simulink model "Correlation_Ex5"  (R2025a)
settings: Solver=VariableStepAuto  StartTime=0.0  StopTime=512/100e6  RelTol=1e-3
InitFcn:
  | RTP_F = 40;
  | RTP_G = 24;
undefined symbols (not defined in the file): Correlation_ValidMode, DUT, Full, S, vsva2197, xcvc1902
libraries: visionstatistics x1, aieDSP x1, aieUtilities x1, vmcUtilities x1
settings Model: Creator=sdegala  LastModifiedBy=sdegala
settings ModelReferenceCC: EnableRefExpFcnMdlSchedulingChecks=on
settings RTWCC: GPUComputeCapability=3.5

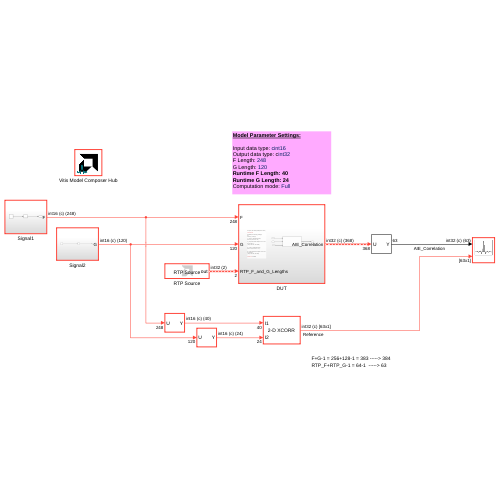
[thumbnail: Simulink's stored preview of the top-level diagram]
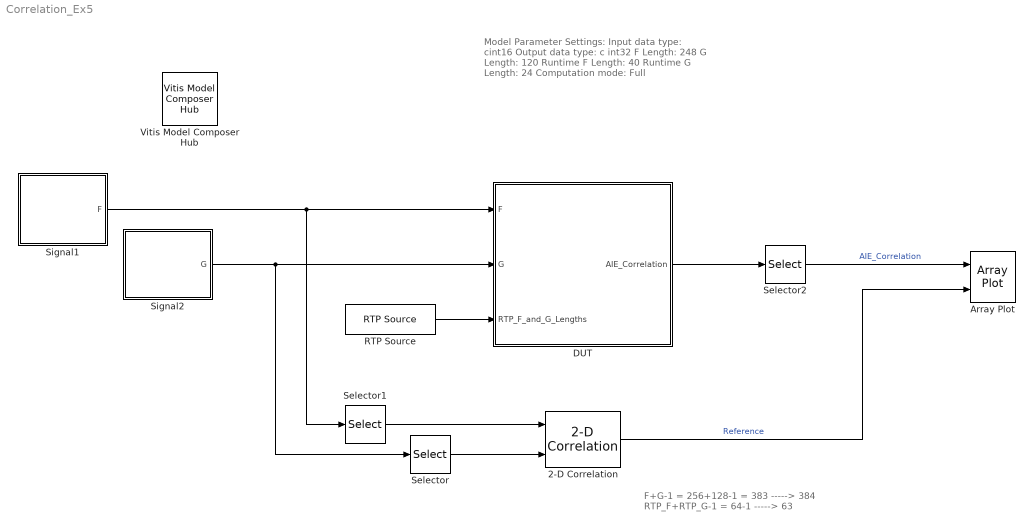
== system Correlation_Ex5 ==
  note: F+G-1 = 256+128-1 = 383 -----> 384
      | RTP_F+RTP_G-1 = 64-1  -----> 63
  note: Model Parameter Settings:
      |
      | Input data type: cint16
      | Output data type: c int32
      | F Length: 248
      | G Length: 120
      | Runtime F Length: 40
      | Runtime G Length: 24
      | Computation mode: Full
  2-D Correlation : visionstatistics/2-D Correlation  outSize=Full  normalize=off  roundingMode=Floor  overflowMode=off  outputMode=Binary point scaling  outputWordLength=32  outputFracLength=0
  Array Plot : ArrayPlot  NumInputPorts=2  WindowPosition=[1138.000000,485.000000,745.000000,420.000000,]  Visible=on  ScopeFrameLocation=window  YLimits=[-15.125 36.125]  ShowLegend=on
  DUT : Subsystem
  RTP Source : aieUtilities/RTP Source  Value=int32([RTP_F,RTP_G]')  SampleTime=-1  OutputForm=Empty
  Selector : Selector  InputPortWidth=120  IndexOptions=Index vector (dialog)  Indices=1:1:RTP_G  OutputSizes=1
  Selector1 : Selector  InputPortWidth=248  IndexOptions=Index vector (dialog)  Indices=1:1:RTP_F  OutputSizes=1
  Selector2 : Selector  InputPortWidth=248+120  IndexOptions=Index vector (dialog)  Indices=1:1:RTP_F+RTP_G-1  OutputSizes=1
  Signal1 : Subsystem
  Signal2 : Subsystem
  Vitis Model Composer Hub : vmcUtilities/Vitis Model Composer Hub  Tag=genX  CodeGeneration=off  SubsystemName=DUT  BlockHierPath=Correlation_ValidMode/DUT  SubsystemType=AIENode  StartColumn=1  NumberOfColumns=1  TargetDirectory=./code  exportDesign=off  analyzeDesign=on  validateDesignOnHw=off  ExportType=AI Engines  IpVendor=xilinx.com  IpLibrary=hls  IpVersion=1.0  IpHWLanguage=Verilog  AieCompilerOptions={}  AieSimulatorOptions={}  CreateTestbench=on  TestbenchStackSize=10  RunRtlSim=off  RunCSim=off  RunAieSim=off  enableSimulationTimeout=on  enableGraphIterations=on  AieSimTimeout=50000  AieGraphIterations=-1  RunAieSimProfiling=off  LaunchVitisAnalyzer=off  PlotOutput=off  RunX86Sim=off  X86SimTimeout=10  GenHwImage=off  GenLibadfXo=off  GenHwValidationCode=off  PlatformType=Not Specified  HwSystemType=Baremetal  HwValidationTarget=hw  ProjDevice=xcvc1902-vsva2197-1LP-e-S  ProjDevicePart=xcvc1902-vsva2197-1LP-e-S  AIEType=AIE  SamplePeriod=-1  ClockFrequency=200  DataPathParallelism=1  xilinxfamily=versalaicore  part=xcvc1902  speed=-1LP-e-S  package=vsva2197  directory=./netlist  testbench=off  incr_netlist=off  synthesis_tool=Vivado  clock_wrapper=Clock Enables  dbl_ovrd=According to Block Masks  dcm_input_clock_period=10  sysclk_period=10  simulink_period=1  eval_field=0  IPInfoJsonString="{\"DUTSubsystemName\":\"DUT\",\"AIESubsystem\":{\"SubsystemName\":\"DUT\",\"TargetDirectory\":\"./code\",\"AIEArrayConfig\":\"Use entire AIE array\",\"StartColumn\":\"0\",\"NumberOfColumns\":\"1\"},\"SubsystemTag\":\"AIENode\"}"  LogFileName=/proj/xhdhdstaff5/sdegala/Head1/HEAD/2025_2_work/AIE_BLOCKS_2025_2/code/model_composer.log  NThreads=4  IPConfigFile=/tmp/vmctmp-11198269997411262707/Correlation_ValidMode_ipconfig.json
  wires:
  Signal1/1(F) -> Selector1/1, DUT/1(F)
  DUT/1(AIE_Correlation) -> Selector2/1
  RTP Source/1 -> DUT/3(RTP_F_and_G_Lengths)
  2-D Correlation/1 -> Array Plot/2  "Reference"
  Selector/1 -> 2-D Correlation/2
  Signal2/1(G) -> DUT/2(G), Selector/1
  Selector1/1 -> 2-D Correlation/1
  Selector2/1 -> Array Plot/1  "AIE_Correlation"

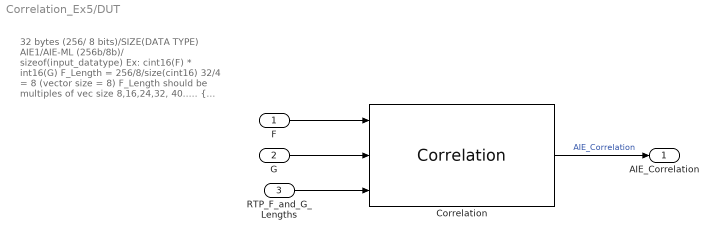
== system Correlation_Ex5/DUT ==
  note: 32 bytes (256/ 8 bits)/SIZE(DATA TYPE)
      |
      | AIE1/AIE-ML
      | (256b/8b)/ sizeof(input_datatype)
      | Ex:
      | cint16(F) * int16(G)
      | F_Length = 256/8/size(cint16)
      | 32/4 = 8 (vector size = 8)
      |
      | F_Length should be multiples of vec size 8,16,24,32, 40.....
      | { range: min-16, max-4096}
      |
      | G_Length = 256/8/size(int16)
      | 32/2 = 16 (vector size = 16)
      |
      | G_Length should be multiples of vec size
      | 16,32,48,64.....
      | { range: min-32, max-256}
      |
      | AIE-MLv2: 512b/8b
  F : Inport
  G : Inport  Port=2
  RTP_F_and_G_Lengths : Inport  Port=3
  Correlation : aieDSP/Correlation  AIE_VARIANT=1  api=0  data_type_f=cint16  data_type_g=cint16  data_type_out=cint32  function_type=0  compute_mode=Full (0)  f_sample_size=248  g_sample_size=120  USE_RTP_VECTOR_LENGTHS=on  num_frames=1  shift_output=0  rnd_mode=Floor  sat_mode=None  no_of_kernels=1  casc_length=1  blockJsonConstraints=[]  blockJsonConstraintsInternal=[]  spec=vmc_corr.json  SerializedMaskParamNames=[]  SerializedMaskParamValues=[]  SerializedMaskParamVisibilities=[]  block_type=Correlation  SerializedMaskParamDataypes=uint|uint|typename|typename|typename|uint|uint|uint|uint|uint|uint|uint|uint|uint|uint|uint  SerializedMaskParamEnumStrArr=0|0|0|0|0|0|Full (0),Same (1),Valid (2)|0|0|0|0|0|Floor,Ceiling,Round to positive infinity,Round to negative infinity,Round symmetrical to infinity,Round symmetrical to zero,Round convergent to even,Round convergent to odd|None,Saturate,Symmetric|0|0  SerializedMaskParamEnumValArr=0|0|0|0|0|0|0,1,2|0|0|0|0|0|0,1,2,3,4,5,6,7|0,1,3|0|0  SerializedMaskParamVectorArr=0|0|0|0|0|0|0|0|0|0|0|0|0|0|0|0  SerializedMaskParamKeys=AIE_VARIANT|TP_API|TT_DATA_F|TT_DATA_G|TT_DATA_OUT|TP_FUNCT_TYPE|TP_COMPUTE_MODE|TP_F_LEN|TP_G_LEN|TP_USE_RTP_VECTOR_LENGTHS|TP_NUM_FRAMES|TP_SHIFT|TP_RND|TP_SAT|TP_PHASES|TP_CASC_LEN
  AIE_Correlation : Outport
  wires:
  F/1 -> Correlation/1
  G/1 -> Correlation/2
  Correlation/1 -> AIE_Correlation/1  "AIE_Correlation"
  RTP_F_and_G_Lengths/1 -> Correlation/3

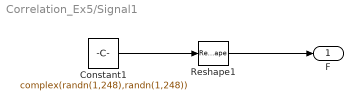
== system Correlation_Ex5/Signal1 ==
  Constant1 : Constant  Value=complex(randn(1,248),randn(1,248))  OutDataTypeStr=int16  SampleTime=1/100e6
  Reshape1 : Reshape
  F : Outport
  wires:
  Reshape1/1 -> F/1
  Constant1/1 -> Reshape1/1

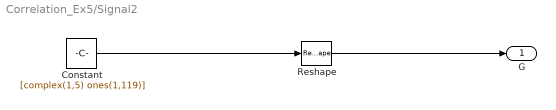
== system Correlation_Ex5/Signal2 ==
  Constant : Constant  Value=[complex(1,5) ones(1,119)]  OutDataTypeStr=int16  SampleTime=1/100e6
  Reshape : Reshape
  G : Outport
  wires:
  Reshape/1 -> G/1
  Constant/1 -> Reshape/1
